simulink model "lqr_cartpend_sim"  (R2019a)
settings: Solver=VariableStepAuto  StartTime=0.0  StopTime=50.0  RelTol=1e-3  EnableMultiTasking=on
undefined symbols (not defined in the file): K
settings Model: Creator=sbrunton  LastModifiedBy=grego
settings DataIOCC: LimitDataPoints=on  ReturnWorkspaceOutputs=off
settings OptimizationCC: LifeSpan=inf
settings DebuggingCC: AllowSymbolicDim=off  SFUnexpectedBacktrackingDiag=warning  SFNoUnconditionalDefaultTransitionDiag=warning  SFExecutionAtInitializationDiag=none  ArithmeticOperatorsInVariantConditions=warning
settings ModelReferenceCC: PropagateSignalLabelsOutOfModel=off
settings SFSimCC: SimUseLocalCustomCode=off
settings RTWCC: RTWUseLocalCustomCode=off
settings CodeAppCC: StateflowObjectComments=on
settings GRTTargetCC: TargetLangStandard=C89/C90 (ANSI)
settings ConfigComp: CovMetricSettings=dw  CovHtmlReporting=on  CovSaveCumulativeToWorkspaceVar=on  CovSaveSingleToWorkspaceVar=on  CovExternalEMLEnable=off

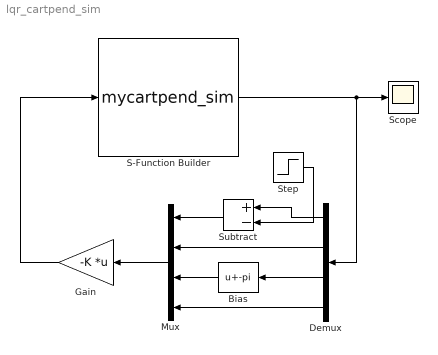
== system lqr_cartpend_sim ==
  Bias : Bias  Bias=-pi
  Demux : Demux
  Gain : Gain  Gain=-K  Multiplication=Matrix(K*u) (u vector)
  Mux : Mux
  S-Function Builder : S-Function  InitFcn=try, set_param(gcb,'FunctionName','mycartpend_sim'), end  FunctionName=mycartpend_sim  SFunctionModules=mycartpend_sim_wrapper  SFunctionDeploymentMode=off  EnableBusSupport=off  mask(S-Function Builder){}
      mask help: Simulink:masks:SFunctionBuilder_MD
      mask init:
      | val = [[.9  0.75 0.75 1 1 .9 .9 1]',[1 1 0.75 0.75 .9 .9 1 .9]'];try , sys = get_param(gcb,'SfunBuilderFcnName');if isempty(sys), sys = get_param(gcb,'FunctionName'); end,catch, sys = get_param(gcb,'FunctionName'); end
      settings: CopyFcn=set_param(gcbh,'LinkStatus','none')  PreSaveFcn=try, set_param(gcb,'FunctionName','mycartpend_sim'), end  OpenFcn=sfunctionwizard(gcbh)
      mask Display: plot(val(:,1),val(:,2)),disp(sys), port_label('input',1,'u0'), port_label('output',1,'y0')
  Scope : Scope
  Step : Step  Time=10  SampleTime=0
  Subtract : Sum  Inputs=+-
  wires:
  Gain/1 -> S-Function Builder/1
  S-Function Builder/1 -> Demux/1, Scope/1
  Demux/2 -> Mux/2
  Demux/4 -> Mux/4
  Demux/3 -> Bias/1
  Bias/1 -> Mux/3
  Mux/1 -> Gain/1
  Subtract/1 -> Mux/1
  Demux/1 -> Subtract/1
  Step/1 -> Subtract/2
